simulink model "Backup"  (R2012b)
settings: Solver=ode45  StartTime=0.0  StopTime=10.0  RelTol=1e-3
settings Model: Creator=David  LastModifiedBy=David

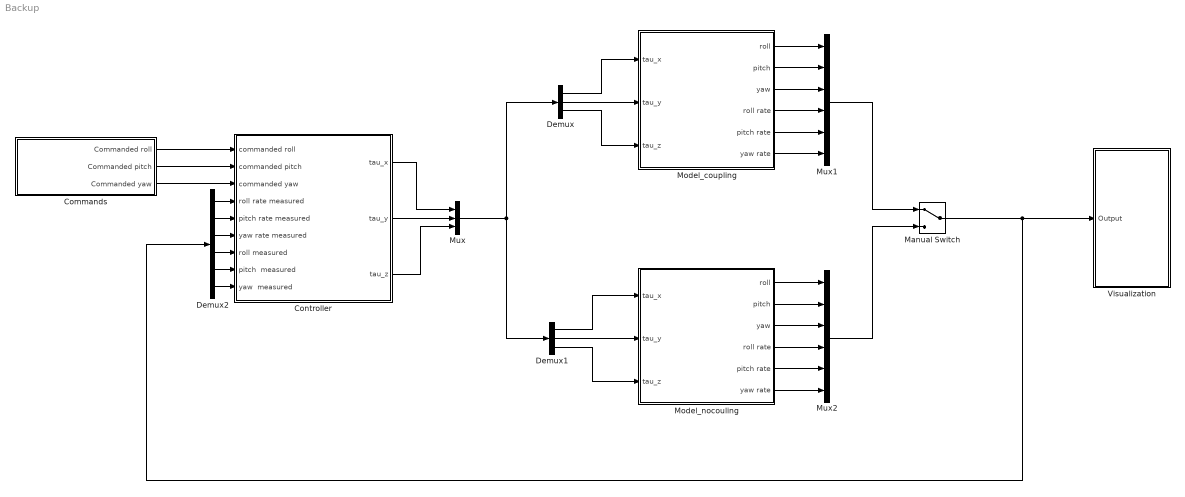
== system Backup ==
  Commands : Subsystem
  Controller : Subsystem
  Demux : Demux  Outputs=3
  Demux1 : Demux  Outputs=3
  Demux2 : Demux  Outputs=6
  Manual Switch : ManualSwitch
  Model_coupling : Subsystem
  Model_nocouling : Subsystem
  Mux : Mux  Inputs=3
  Mux1 : Mux  Inputs=6
  Mux2 : Mux  Inputs=6
  Visualization : Subsystem
  wires:
  Controller/1("tau_x ") -> Mux/1
  Controller/2(tau_y) -> Mux/2
  Controller/3(tau_z) -> Mux/3
  Demux/1 -> Model_coupling/1(tau_x)
  Demux/2 -> Model_coupling/2(tau_y)
  Demux/3 -> Model_coupling/3(tau_z)
  Demux1/1 -> Model_nocouling/1(tau_x)
  Demux1/2 -> Model_nocouling/2(tau_y)
  Demux1/3 -> Model_nocouling/3(tau_z)
  Model_coupling/1(roll) -> Mux1/1
  Model_coupling/2(pitch) -> Mux1/2
  Model_coupling/3(yaw) -> Mux1/3
  Model_coupling/4(roll rate) -> Mux1/4
  Model_coupling/5(pitch rate) -> Mux1/5
  Model_coupling/6(yaw rate) -> Mux1/6
  Model_nocouling/1(roll) -> Mux2/1
  Model_nocouling/2(pitch) -> Mux2/2
  Model_nocouling/3(yaw) -> Mux2/3
  Model_nocouling/4(roll rate) -> Mux2/4
  Model_nocouling/5(pitch rate) -> Mux2/5
  Model_nocouling/6(yaw rate) -> Mux2/6
  Mux1/1 -> Manual Switch/1
  Mux2/1 -> Manual Switch/2
  Mux/1 -> Demux/1, Demux1/1
  Manual Switch/1 -> Visualization/1(Output), Demux2/1
  Demux2/1 -> Controller/4(roll rate measured)
  Demux2/2 -> Controller/5(pitch rate measured)
  Demux2/3 -> Controller/6(yaw rate measured)
  Demux2/4 -> Controller/7(roll measured)
  Demux2/5 -> Controller/8(pitch  measured)
  Demux2/6 -> Controller/9(yaw  measured)
  Commands/1(Commanded roll) -> Controller/1(commanded roll)
  Commands/2(Commanded pitch) -> Controller/2(commanded pitch)
  Commands/3(Commanded yaw) -> Controller/3(commanded yaw)

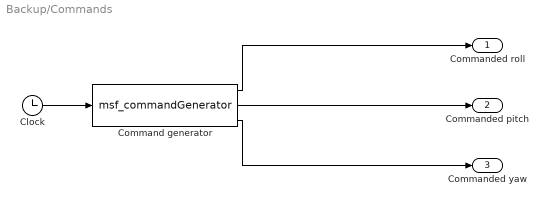
== system Backup/Commands ==
  Clock : Clock
  Command generator : M-S-Function  FunctionName=msf_commandGenerator  Parameters=0.1
  Commanded roll : Outport
  Commanded pitch : Outport  Port=2
  Commanded yaw : Outport  Port=3
  wires:
  Command generator/1 -> Commanded roll/1
  Command generator/2 -> Commanded pitch/1
  Command generator/3 -> Commanded yaw/1
  Clock/1 -> Command generator/1

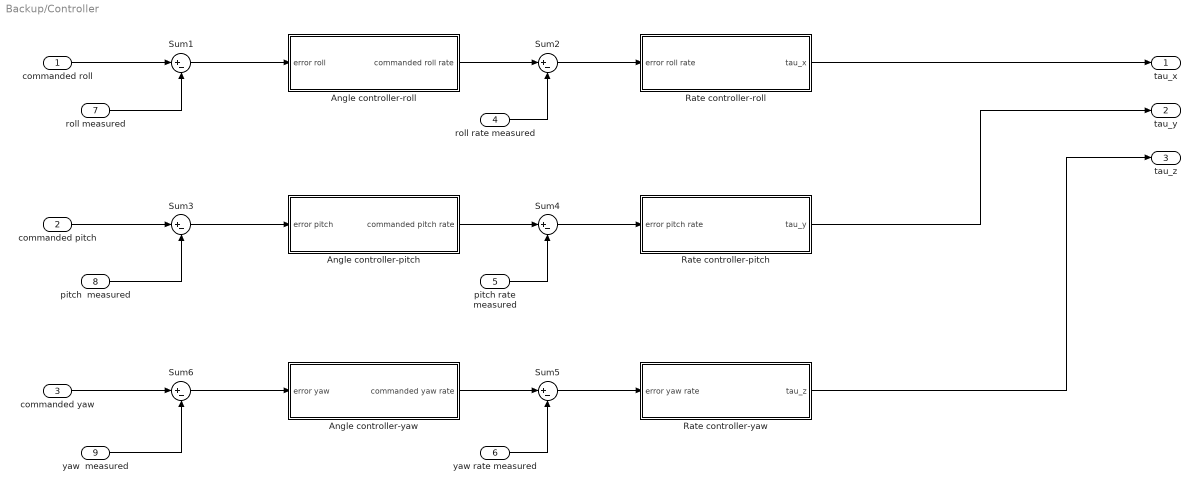
== system Backup/Controller ==
  commanded roll : Inport
  commanded pitch : Inport  Port=2
  commanded yaw : Inport  Port=3
  roll rate measured : Inport  Port=4
  pitch rate measured : Inport  Port=5
  yaw rate measured : Inport  Port=6
  roll measured : Inport  Port=7
  pitch  measured : Inport  Port=8
  yaw  measured : Inport  Port=9
  Angle controller-pitch : Subsystem
  Angle controller-roll : Subsystem
  Angle controller-yaw : Subsystem
  Rate controller-pitch : Subsystem
  Rate controller-roll : Subsystem
  Rate controller-yaw : Subsystem
  Sum{1..6} (6 alike) : Sum  Inputs=|+-
  "tau_x " : Outport
  tau_y : Outport  Port=2
  tau_z : Outport  Port=3
  wires:
  Sum1/1 -> Angle controller-roll/1(error roll)
  commanded roll/1 -> Sum1/1
  roll measured/1 -> Sum1/2
  roll rate measured/1 -> Sum2/2
  Angle controller-roll/1(commanded roll rate) -> Sum2/1
  Sum2/1 -> Rate controller-roll/1(error roll rate)
  commanded pitch/1 -> Sum3/1
  Sum3/1 -> Angle controller-pitch/1(error pitch)
  pitch  measured/1 -> Sum3/2
  Angle controller-pitch/1(commanded pitch rate) -> Sum4/1
  pitch rate measured/1 -> Sum4/2
  Sum4/1 -> Rate controller-pitch/1(error pitch rate)
  commanded yaw/1 -> Sum6/1
  yaw  measured/1 -> Sum6/2
  Sum6/1 -> Angle controller-yaw/1(error yaw)
  Angle controller-yaw/1(commanded yaw rate) -> Sum5/1
  yaw rate measured/1 -> Sum5/2
  Sum5/1 -> Rate controller-yaw/1(error yaw rate)
  Rate controller-roll/1(tau_x) -> "tau_x "/1
  Rate controller-pitch/1(tau_y) -> tau_y/1
  Rate controller-yaw/1(tau_z) -> tau_z/1

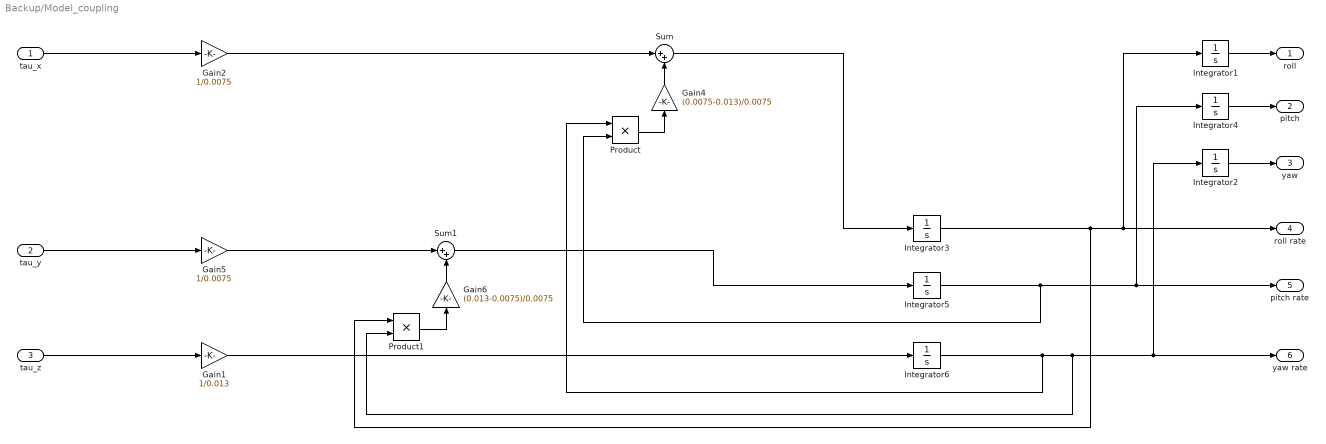
== system Backup/Model_coupling ==
  tau_x : Inport
  tau_y : Inport  Port=2
  tau_z : Inport  Port=3
  Gain1 : Gain  Gain=1/0.013
  Gain2 : Gain  Gain=1/0.0075
  Gain4 : Gain  Gain=(0.0075-0.013)/0.0075
  Gain5 : Gain  Gain=1/0.0075
  Gain6 : Gain  Gain=(0.013-0.0075)/0.0075
  Integrator{1..6} (6 alike) : Integrator
  Product : Product  RndMeth=Zero
  Product1 : Product  RndMeth=Zero
  Sum : Sum  Inputs=|++
  Sum1 : Sum  Inputs=|++
  roll : Outport
  pitch : Outport  Port=2
  yaw : Outport  Port=3
  roll rate : Outport  Port=4
  pitch rate : Outport  Port=5
  yaw rate : Outport  Port=6
  wires:
  Integrator1/1 -> roll/1
  Integrator4/1 -> pitch/1
  Integrator2/1 -> yaw/1
  Integrator3/1 -> Product1/1, roll rate/1, Integrator1/1
  Integrator5/1 -> Integrator4/1, pitch rate/1, Product/2
  Integrator6/1 -> Product/1, Product1/2, Integrator2/1, yaw rate/1
  Product/1 -> Gain4/1
  Gain2/1 -> Sum/1
  Gain4/1 -> Sum/2
  tau_x/1 -> Gain2/1
  Sum/1 -> Integrator3/1
  Product1/1 -> Gain6/1
  Gain5/1 -> Sum1/1
  Gain6/1 -> Sum1/2
  tau_y/1 -> Gain5/1
  Sum1/1 -> Integrator5/1
  tau_z/1 -> Gain1/1
  Gain1/1 -> Integrator6/1

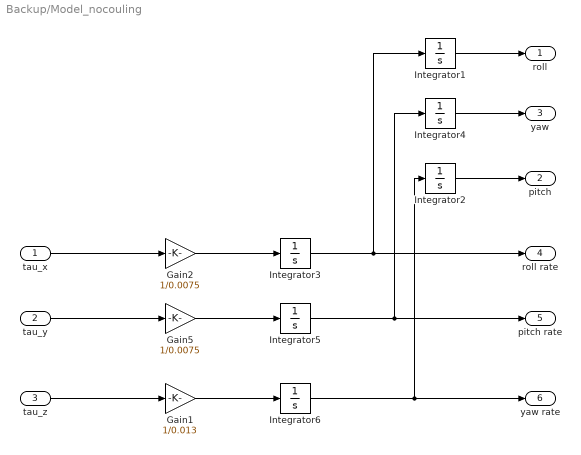
== system Backup/Model_nocouling ==
  tau_x : Inport
  tau_y : Inport  Port=2
  tau_z : Inport  Port=3
  Gain1 : Gain  Gain=1/0.013
  Gain2 : Gain  Gain=1/0.0075
  Gain5 : Gain  Gain=1/0.0075
  Integrator{1..6} (6 alike) : Integrator
  roll : Outport
  pitch : Outport  Port=2
  yaw : Outport  Port=3
  roll rate : Outport  Port=4
  pitch rate : Outport  Port=5
  yaw rate : Outport  Port=6
  wires:
  Integrator3/1 -> roll rate/1, Integrator1/1
  Integrator5/1 -> pitch rate/1, Integrator4/1
  Integrator6/1 -> yaw rate/1, Integrator2/1
  Gain1/1 -> Integrator6/1
  Gain2/1 -> Integrator3/1
  Gain5/1 -> Integrator5/1
  tau_x/1 -> Gain2/1
  tau_y/1 -> Gain5/1
  tau_z/1 -> Gain1/1
  Integrator1/1 -> roll/1
  Integrator4/1 -> yaw/1
  Integrator2/1 -> pitch/1

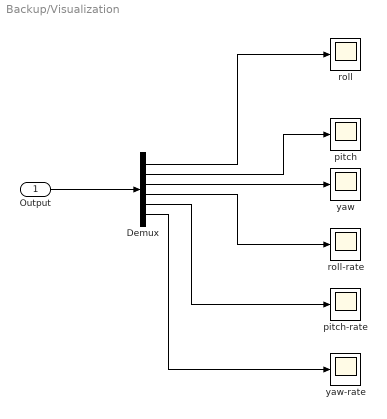
== system Backup/Visualization ==
  Output : Inport
  Demux : Demux  Outputs=6
  pitch : Scope
      settings: SaveName=pitch
  pitch-rate : Scope
      settings: TimeRange=10  SaveName=pitch_rate
  roll : Scope
      settings: TimeRange=10  SaveName=roll
  roll-rate : Scope
      settings: TimeRange=10  SaveName=roll_rate
  yaw : Scope
      settings: SaveName=yaw
  yaw-rate : Scope
      settings: TimeRange=10  SaveName=yaw_rate
  wires:
  Output/1 -> Demux/1
  Demux/1 -> roll/1
  Demux/2 -> pitch/1
  Demux/3 -> yaw/1
  Demux/4 -> roll-rate/1
  Demux/5 -> pitch-rate/1
  Demux/6 -> yaw-rate/1

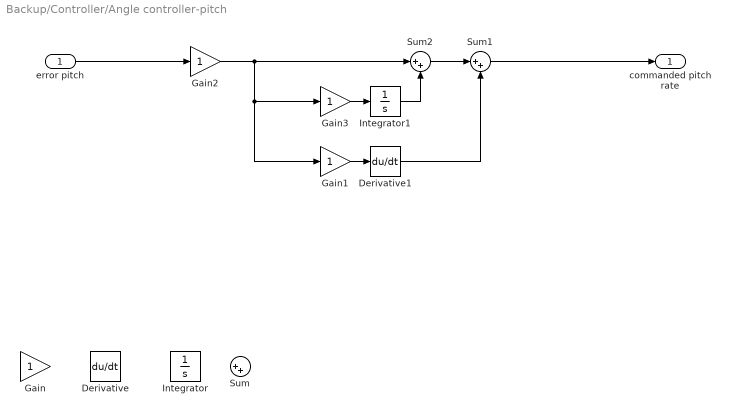
== system Backup/Controller/Angle controller-pitch ==
  error pitch : Inport
  Derivative : Derivative
  Derivative1 : Derivative
  Gain{,1..3} (4 alike) : Gain
  Integrator : Integrator
  Integrator1 : Integrator
  Sum : Sum  Inputs=|++
  Sum1 : Sum  Inputs=|++
  Sum2 : Sum  Inputs=|++
  commanded pitch rate : Outport
  wires:
  Integrator1/1 -> Sum2/2
  Gain2/1 -> Gain1/1, Gain3/1, Sum2/1
  Gain3/1 -> Integrator1/1
  Sum2/1 -> Sum1/1
  Derivative1/1 -> Sum1/2
  Gain1/1 -> Derivative1/1
  error pitch/1 -> Gain2/1
  Sum1/1 -> commanded pitch rate/1

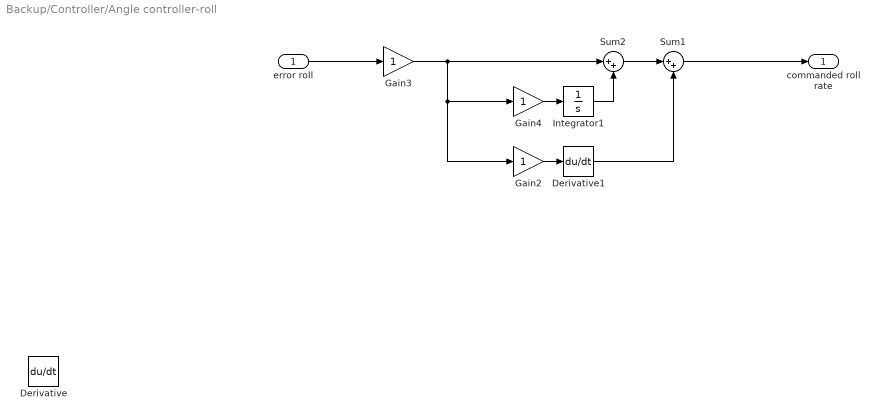
== system Backup/Controller/Angle controller-roll ==
  error roll : Inport
  Derivative : Derivative
  Derivative1 : Derivative
  Gain2 : Gain
  Gain3 : Gain
  Gain4 : Gain
  Integrator1 : Integrator
  Sum1 : Sum  Inputs=|++
  Sum2 : Sum  Inputs=|++
  commanded roll rate : Outport
  wires:
  Integrator1/1 -> Sum2/2
  Gain3/1 -> Gain2/1, Gain4/1, Sum2/1
  Gain4/1 -> Integrator1/1
  Sum2/1 -> Sum1/1
  Derivative1/1 -> Sum1/2
  Gain2/1 -> Derivative1/1
  error roll/1 -> Gain3/1
  Sum1/1 -> commanded roll rate/1

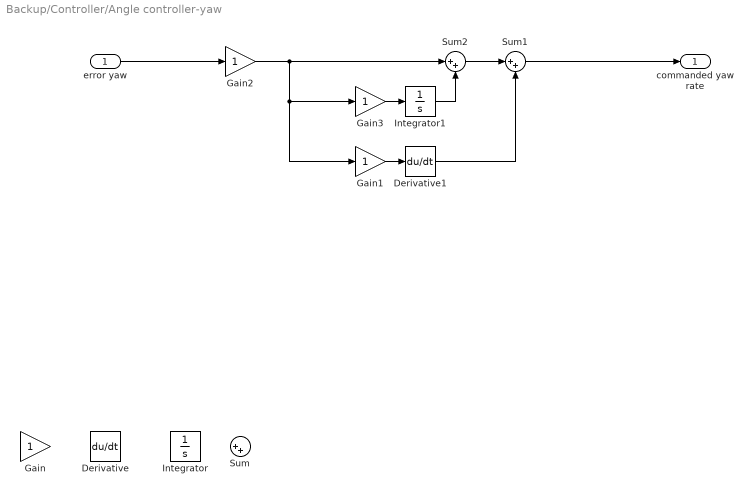
== system Backup/Controller/Angle controller-yaw ==
  error yaw : Inport
  Derivative : Derivative
  Derivative1 : Derivative
  Gain{,1..3} (4 alike) : Gain
  Integrator : Integrator
  Integrator1 : Integrator
  Sum : Sum  Inputs=|++
  Sum1 : Sum  Inputs=|++
  Sum2 : Sum  Inputs=|++
  commanded yaw rate : Outport
  wires:
  Integrator1/1 -> Sum2/2
  Gain2/1 -> Gain1/1, Gain3/1, Sum2/1
  Gain3/1 -> Integrator1/1
  Sum2/1 -> Sum1/1
  Derivative1/1 -> Sum1/2
  Gain1/1 -> Derivative1/1
  error yaw/1 -> Gain2/1
  Sum1/1 -> commanded yaw rate/1

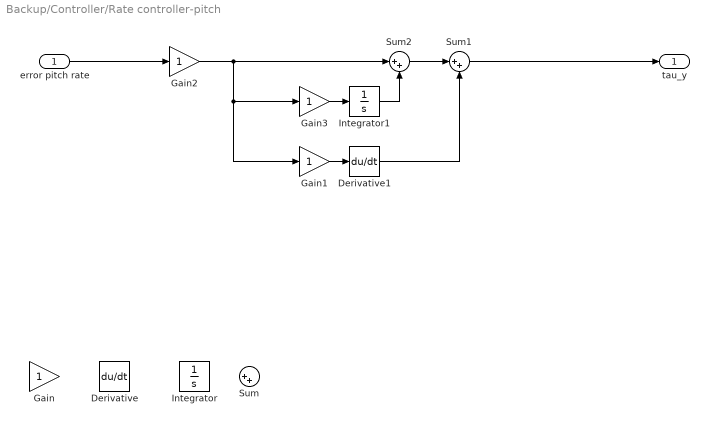
== system Backup/Controller/Rate controller-pitch ==
  error pitch rate : Inport
  Derivative : Derivative
  Derivative1 : Derivative
  Gain{,1..3} (4 alike) : Gain
  Integrator : Integrator
  Integrator1 : Integrator
  Sum : Sum  Inputs=|++
  Sum1 : Sum  Inputs=|++
  Sum2 : Sum  Inputs=|++
  tau_y : Outport
  wires:
  Integrator1/1 -> Sum2/2
  Gain2/1 -> Gain1/1, Gain3/1, Sum2/1
  Gain3/1 -> Integrator1/1
  Sum2/1 -> Sum1/1
  Derivative1/1 -> Sum1/2
  Gain1/1 -> Derivative1/1
  error pitch rate/1 -> Gain2/1
  Sum1/1 -> tau_y/1

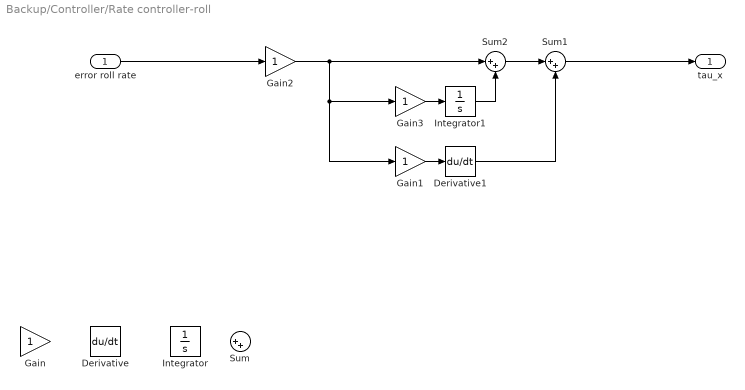
== system Backup/Controller/Rate controller-roll ==
  error roll rate : Inport
  Derivative : Derivative
  Derivative1 : Derivative
  Gain{,1..3} (4 alike) : Gain
  Integrator : Integrator
  Integrator1 : Integrator
  Sum : Sum  Inputs=|++
  Sum1 : Sum  Inputs=|++
  Sum2 : Sum  Inputs=|++
  tau_x : Outport
  wires:
  Integrator1/1 -> Sum2/2
  Gain2/1 -> Gain1/1, Gain3/1, Sum2/1
  Gain3/1 -> Integrator1/1
  Sum2/1 -> Sum1/1
  Derivative1/1 -> Sum1/2
  Gain1/1 -> Derivative1/1
  error roll rate/1 -> Gain2/1
  Sum1/1 -> tau_x/1

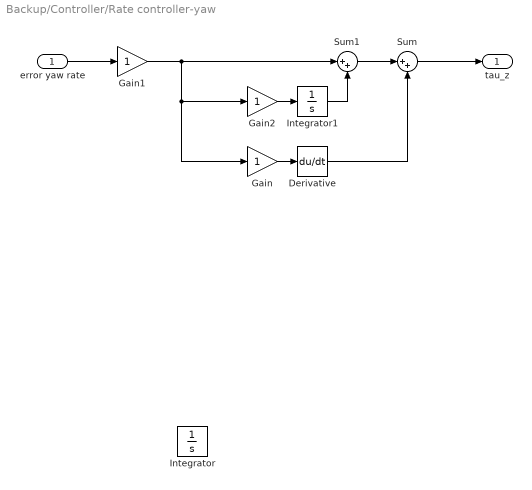
== system Backup/Controller/Rate controller-yaw ==
  error yaw rate : Inport
  Derivative : Derivative
  Gain : Gain
  Gain1 : Gain
  Gain2 : Gain
  Integrator : Integrator
  Integrator1 : Integrator
  Sum : Sum  Inputs=|++
  Sum1 : Sum  Inputs=|++
  tau_z : Outport
  wires:
  Integrator1/1 -> Sum1/2
  Gain1/1 -> Gain/1, Gain2/1, Sum1/1
  Gain2/1 -> Integrator1/1
  error yaw rate/1 -> Gain1/1
  Sum1/1 -> Sum/1
  Derivative/1 -> Sum/2
  Sum/1 -> tau_z/1
  Gain/1 -> Derivative/1
